simulink model "MPC_AVC_implementation"  (Simulink 7.1)
settings: Solver=ode5  StartTime=0.0  StopTime=Total_t_sim  FixedStep=dt  RelTol=1e-3
PostLoadFcn:
  | , if any(exist('dsrtsu_mdlpostloadfcn', 'file') == [2, 3, 6]), try dsrtsu_mdlpostloadfcn('Execute', bdroot); catch fprintf('Error in PostLoadFcn (dsrtsu_mdlpostloadfcn) for model "%s":\n %s\n', bdroot, lasterr); end, end,
undefined symbols (not defined in the file or in its folder): A, A_cons, Ag, B, Bg, C, coefs, dt, Hg, L_m, Lf, omega, Ps, psi, Rs, Total_t_sim, u_bound
libraries: simulink x3, dsparch4 x1, rti2004lib x1, rtilibm x1
settings Model: Creator=durranbm  LastModifiedBy=oveisahw  BufferReuse=off  DSRTSU_INTERNAL_RTI_VER=330  DSRTSU_INTERNAL_RTI_TYPE=rti1005
settings SolverCC: AlgebraicLoopSolver=LineSearch
settings OptimizationCC: BlockReduction=off  OptimizeBlockIOStorage=off  BufferReuse=off  ExpressionFolding=off  LocalBlockOutputs=off
settings DebuggingCC: AlgebraicLoopMsg=none  ArtificialAlgebraicLoopMsg=none
settings HardwareCC: ProdIntDivRoundTo=Zero  ProdEndianess=BigEndian  ProdHWDeviceType=Specified  TargetIntDivRoundTo=Zero  TargetEndianess=BigEndian
settings RTWCC: SystemTargetFile=rti1005.tlc  MakeCommand=make_rti  TemplateMakefile=rti1005.tmf  Description=dSPACE DS1005 Hardware Platform  ProcessScript=rti1005_make_rtw_hook
settings STFCustomTargetCC: SystemTargetFile=rti1005.tlc
settings GRTTargetCC: CompOptLevelCompliant=off  MatFileLogging=off  ExtModeMexFile=noextcomm
settings CustomProperty: DataType=RTWOptions_EnumType_C__dSPACE_matlab_rti1005_tlc_rti1005_InitialSimState  Value=RUN
settings EnumStrPairs: String=RUN

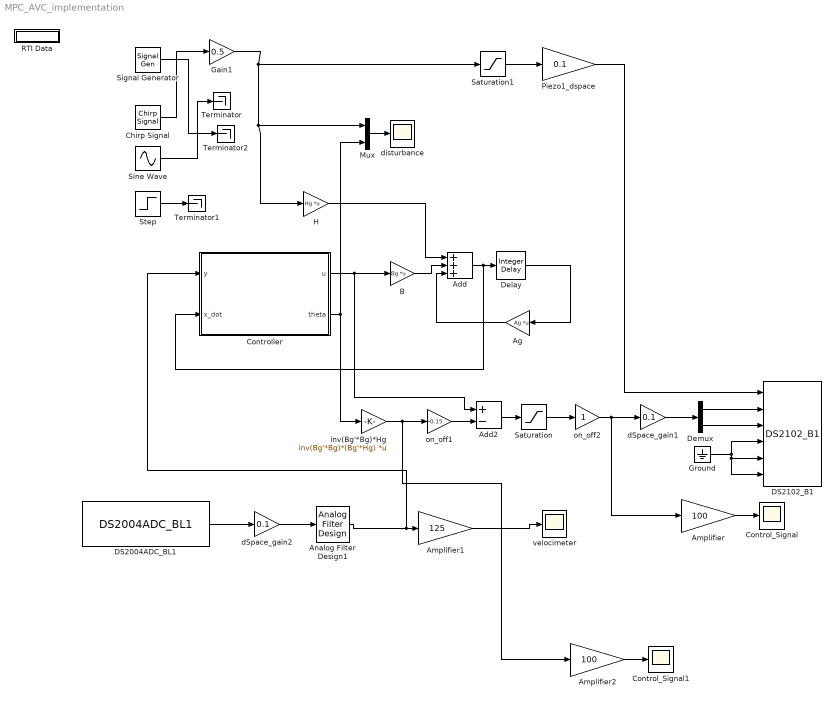
== system MPC_AVC_implementation ==
  Add : Sum  Inputs=+++
  Add2 : Sum  Inputs=+-
  Ag : Gain  Orientation=left  Gain=Ag  Multiplication=Matrix(K*u)
  Amplifier : Gain  Gain=100  ParameterDataType=sfix(16)  ParameterScaling=2^0  OutDataType=sfix(16)  OutScaling=2^0
  Amplifier1 : Gain  Gain=125  ParameterDataType=sfix(16)  ParameterScaling=2^0  OutDataType=sfix(16)  OutScaling=2^0
  Amplifier2 : Gain  Gain=100  ParameterDataType=sfix(16)  ParameterScaling=2^0  OutDataType=sfix(16)  OutScaling=2^0
  Analog Filter Design1 : dsparch4/Analog Filter Design  method=Butterworth  filttype=Lowpass  N=4  Wlo=(2*pi)*400  Whi=80  Rp=2  Rs=40
  B : Gain  Gain=Bg  Multiplication=Matrix(K*u)
  Chirp Signal : simulink/Sources/Chirp Signal  SystemSampleTime=-1  f1=1  T=Total_t_sim  f2=90
  Control_Signal : Scope
      settings: YMin=-1  YMax=1  SaveName=ScopeData2  MaxDataPoints=500000
  Control_Signal1 : Scope
      settings: YMin=-1  YMax=1  SaveName=ScopeData3  MaxDataPoints=500000
  Controller : Subsystem
  DS2004ADC_BL1 : rti2004lib/DS2004ADC_BL1  SystemSampleTime=-1  DSProperties=struct('RTI',struct('Version',uint32(1),'BlockType',struct('isSLSource',uint8(1),'isSLSink',uint8(1),'isHWSource',uint8(0),'isHWSink',uint8(1),'isSetup',uint8(0),'isInline',uint8(1),'isNonInline',uint8(0),'isInterrupt',uint8(0),'isChannelwise',uint8(1)),'IOBoardType','DS2004','UnitType','ADC','Identifier','ADC','DialogType','ML','BlockSet','NONE','SlaveProcessor','NONE'))  RTIBlockInterface=struct('InputPortsActive',0,'InputPortsWidth',int32(1),'InputPortsDataType',{{'SS_BOOLEAN'}},'InputPortsName',{{'Continue'}},'OutputPortsActive',[1 0],'OutputPortsWidth',int32([1 1]),'OutputPortsDataType',{{'SS_DOUBLE','SS_UINT8'}},'OutputPortsName',{{'ADC','Status'}},'DialogFcn','rti2004adcgui','SampleTime',{{-1}},'InitLevel',3,'IconTransparency','on','BlockDisplay',{{['DS2004 ADC\nBoard: 1\nChannel: 1'],'center'}},'BlockName',struct('Token',{{'DS2004ADC_BL1'}}))  RTIBlockParameters=struct('ADCSWStartDisable',{{0,'OFF',[0 1]}},'BoardNo',{{1,'OFF',[1 16]}},'ChannelNo',{{1,'OFF',[1 16]}},'ConversionMode',{{1,'OFF',[1 2]}},'SampleMode',{{1,'OFF',[1 2]}},'TriggerSource',{{1,'OFF',[1 5]}},'EdgePolarity',{{1,'OFF',[1 2]}},'ConversionTriggerSource',{{2,'OFF',[1 6]}},'ConversionEdgePolarity',{{1,'OFF',[1 2]}},'ConversionPeriod',{{'1e-006','OFF',[]}},'ConversionPeriodCheck',{{0,'OFF',[]}},'BurstTriggerSource',{{1,'OFF',[1 6]}},'BurstEdgePolarity',{{1,'OFF',[1 2]}},'BurstSize',{{'10','OFF',[]}},'BurstSizeCheck',{{0,'OFF',[]}},'DataSetOffset',{{'0','OFF',[]}},'DataSetOffsetCheck',{{0,'OFF',[]}},'DataSetLength',{{'1','OFF',[]}},'DataSetLengthCheck',{{0,'OFF',[]}},'ReadMode',{{1,'OFF',[1 2]}},'SampleTime',{{'-1','OFF',[-1 inf]}},'SampleTimeCheck',{{1,'OFF',[]}},'InputVoltageRange',{{2,'OFF',[1 2]}},'StatusPortEnable',{{0,'OFF',[0 1]}},'TLCFileName',{{'rti2004adc','OFF',[]}})  RTISFcnParameters=struct('ADCSWStartDisable','int32','BoardNo','int32','ChannelNo','int32','ConversionMode','int32','SampleMode','int32','TriggerSource','int32','EdgePolarity','int32','ConversionTriggerSource','int32','ConversionEdgePolarity','int32','ConversionPeriod','double','BurstTriggerSource','int32','BurstEdgePolarity','int32','BurstSize','int32','DataSetOffset','int32','DataSetLength','int32','ReadMode','int32','SampleTime','double','InputVoltageRange','int32','StatusPortEnable','int32','TLCFileName','char')  RTIBlockParaDefault=struct('ADCSWStartDisable',0,'BoardNo',1,'ChannelNo',1,'ConversionMode',1,'SampleMode',1,'TriggerSource',1,'EdgePolarity',1,'ConversionTriggerSource',2,'ConversionEdgePolarity',1,'ConversionPeriod',1e-06,'ConversionPeriodCheck',0,'BurstTriggerSource',1,'BurstEdgePolarity',1,'BurstSize',10,'BurstSizeCheck',0,'DataSetOffset',0,'DataSetOffsetCheck',0,'DataSetLength',1,'DataSetLengthCheck',0,'ReadMode',1,'SampleTime',-1,'SampleTimeCheck',1,'InputVoltageRange',2,'StatusPortEnable',0,'TLCFileName','rti2004adc')
  DS2102_B1 : rtilibm/DS2102/DS2102_B1  SystemSampleTime=-1  BoardNo=1  Range=[10 10 10 10 10 10]  IOErrorMode=[1 1 1 1 1 1]  DeglitcherMode=[0 0 0 0 0 0]  InitValue=[0 0 0 0 0 0]  TermMode=[1 1 1 1 1 1]  TermValue=[0 0 0 0 0 0]  DialogFcn=gui2102  UnitName={'DS2102_B'}  UnitValues={ 1 }  DSProperties=struct('RTI',struct('Version',uint32(1),'BlockType',struct('isSLSource',uint8(0),'isSLSink',uint8(1),'isHWSource',uint8(0),'isHWSink',uint8(1),'isSetup',uint8(0),'isInline',uint8(1),'isNonInline',uint8(0),'isInterrupt',uint8(0),'isChannelwise',uint8(0)),'IOBoardType','DS2102','UnitType','DAC','Identifier','DAC','DialogType','ML','BlockSet','NONE','SlaveProcessor','NONE'))
  Delay : simulink/Discrete/Integer Delay  vinit=0  samptime=-1  NumDelays=1
  Demux : Demux  Outputs=2
  Gain1 : Gain  Gain=0.5  ParameterDataType=sfix(16)  ParameterScaling=2^0  OutDataType=sfix(16)  OutScaling=2^0
  Ground : Ground
  H : Gain  Gain=Hg  Multiplication=Matrix(K*u)
  Mux : Mux  Inputs=2
  Piezo1_dspace : Gain  Gain=0.1  ParameterDataType=sfix(16)  ParameterScaling=2^0  OutDataType=sfix(16)  OutScaling=2^0
  RTI Data : Subsystem  Tag=struct('RTIDataServer',struct('RTIDataServerVs','2','RTIModelDescription','struct(''main'',''MPC_AVC_implementation'',''sub'','''',''isMp'',0)'))  LoadFcn="if exist('rtidc'), try,  rtidc('DataHostBlockClbLoad', gcbh); catch, disp(['Warning: ''LoadFcn'' for RTI Data block failed: ' lasterr]); end, end,"
      settings: CopyFcn="if exist('rtidc'), try,  rtidc('DataHostBlockClbCopy', gcbh); catch, disp(['Warning: ''CopyFcn'' for RTI Data block failed: ' lasterr]); end, end,"  DeleteFcn="if exist('rtidc'), try,  rtidc('DataHostBlockClbDelete', gcbh); catch, disp(['Warning: ''DeleteFcn'' for RTI Data block failed: ' lasterr]); end, end,"  ModelCloseFcn="if exist('rtidc'), try,  rtidc('DataHostBlockClbModelClose', gcbh); catch, disp(['Warning: ''ModelCloseFcn'' for RTI Data block failed: ' lasterr]); end, end,"  PreSaveFcn="if exist('rtidc'), try,  rtidc('DataHostBlockClbPreSave', gcbh); catch, disp(['Warning: ''PreSaveFcn'' for RTI Data block failed: ' lasterr]); end, end,"  PostSaveFcn="if exist('rtidc'), try,  rtidc('DataHostBlockClbPostSave', gcbh); catch, disp(['Warning: ''PostSaveFcn'' for RTI Data block failed: ' lasterr]); end, end,"  NameChangeFcn="if exist('rtidc'), try,  rtidc('DataHostBlockClbNameChange', gcbh); catch, disp(['Warning: ''NameChangeFcn'' for RTI Data block failed: ' lasterr]); end, end,"
      mask Type: RTI_DATA_HOST
      mask Description:
      | RTI Data Block.
      | This block is used by RTI to store internal model-dependent data.
      | Please keep this block on the root level of the model. Deleting this block will result in data loss.
      | 
      | NEVER DELETE OR COPY THIS BLOCK!
      mask Help:
      | RTI Data Block.
      | This block is used by RTI to store internal model-dependent data.
      | Please keep this block on the root level of the model. Deleting this block will result in data loss.
      | 
      | NEVER DELETE OR COPY THIS BLOCK!
      mask Display:
      | text(0.5, 0.5, 'RTI Data', 'HorizontalAlignment', 'center');
      | plot([1 0]);
  Saturation : Saturate  UpperLimit=2  LowerLimit=-2  OutDataType=sfix(16)  OutScaling=2^0
  Saturation1 : Saturate  UpperLimit=1  LowerLimit=-1  OutDataType=sfix(16)  OutScaling=2^0
  Signal Generator : SignalGenerator  WaveForm=square  Frequency=1/2.5
  Sine Wave : Sin  Frequency=71*2*pi  SampleTime=dt
  Step : Step  Time=2*dt  SampleTime=0
  Terminator : Terminator
  Terminator1 : Terminator
  Terminator2 : Terminator
  dSpace_gain1 : Gain  Gain=0.1  ParameterDataType=sfix(16)  ParameterScaling=2^0  OutDataType=sfix(16)  OutScaling=2^0
  dSpace_gain2 : Gain  Gain=0.1  ParameterDataType=sfix(16)  ParameterScaling=2^0  OutDataType=sfix(16)  OutScaling=2^0
  disturbance : Scope
      settings: YMin=-0.0007  YMax=0.0007  SaveName=ScopeData5
  inv(Bg'*Bg)*Hg : Gain  Gain=inv(Bg'*Bg)*(Bg'*Hg)  Multiplication=Matrix(K*u)
  on_off1 : Gain  Gain=-0.15
  on_off2 : Gain
  velocimeter : Scope
  wires:
  DS2004ADC_BL1/1 -> dSpace_gain2/1
  dSpace_gain2/1 -> Analog Filter Design1/1
  Amplifier/1 -> Control_Signal/1
  Saturation/1 -> on_off2/1
  on_off2/1 -> Amplifier/1, dSpace_gain1/1
  Step/1 -> Terminator1/1
  dSpace_gain1/1 -> Demux/1
  Demux/1 -> DS2102_B1/2
  Demux/2 -> DS2102_B1/3
  Ground/1 -> DS2102_B1/5, DS2102_B1/6, DS2102_B1/4
  Saturation1/1 -> Piezo1_dspace/1
  Piezo1_dspace/1 -> DS2102_B1/1
  Controller/1(u) -> B/1, Add2/1
  Delay/1 -> Ag/1
  Add/1 -> Controller/2(x_dot), Delay/1
  Ag/1 -> Add/3
  H/1 -> Add/1
  B/1 -> Add/2
  Add2/1 -> Saturation/1
  inv(Bg'*Bg)*Hg/1 -> Amplifier2/1, on_off1/1
  Amplifier1/1 -> velocimeter/1
  Controller/2(theta) -> inv(Bg'*Bg)*Hg/1, Mux/2
  Analog Filter Design1/1 -> Controller/1(y), Amplifier1/1
  Amplifier2/1 -> Control_Signal1/1
  on_off1/1 -> Add2/2
  Sine Wave/1 -> Terminator/1
  Mux/1 -> disturbance/1
  Signal Generator/1 -> Terminator2/1
  Chirp Signal/1 -> Gain1/1
  Gain1/1 -> Saturation1/1, H/1, Mux/1

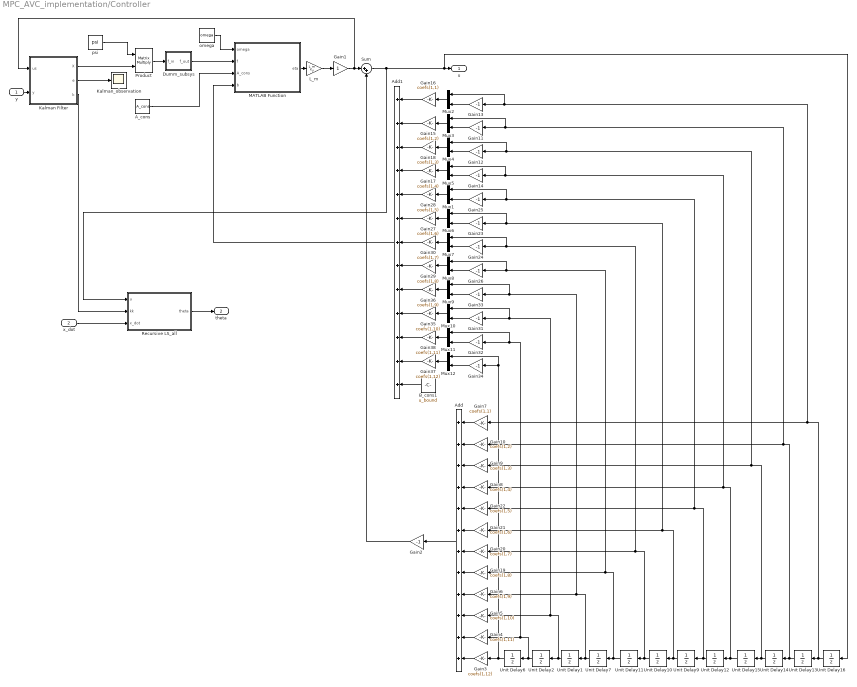
== system MPC_AVC_implementation/Controller ==
  y : Inport
  x_dot : Inport  Port=2
  A_cons : Constant  Value=A_cons  SampleTime=dt
  Add : Sum  Orientation=left  Inputs=++++++++++++
  Add1 : Sum  Orientation=left  Inputs=+++++++++++++
  B_cons1 : Constant  Orientation=left  Value=u_bound
  Dumm_subsys : Subsystem
  Gain1 : Gain
  Gain10 : Gain  Orientation=left  Gain=coefs(1,2)
  Gain{2,11..14,23..26,31..34} (13 alike) : Gain  Orientation=left  Gain=-1
  Gain15 : Gain  Orientation=left  Gain=coefs(1,2)
  Gain16 : Gain  Orientation=left  Gain=coefs(1,1)
  Gain17 : Gain  Orientation=left  Gain=coefs(1,4)
  Gain18 : Gain  Orientation=left  Gain=coefs(1,3)
  Gain19 : Gain  Orientation=left  Gain=coefs(1,8)
  Gain20 : Gain  Orientation=left  Gain=coefs(1,7)
  Gain21 : Gain  Orientation=left  Gain=coefs(1,6)
  Gain22 : Gain  Orientation=left  Gain=coefs(1,5)
  Gain27 : Gain  Orientation=left  Gain=coefs(1,6)
  Gain28 : Gain  Orientation=left  Gain=coefs(1,5)
  Gain29 : Gain  Orientation=left  Gain=coefs(1,8)
  Gain3 : Gain  Orientation=left  Gain=coefs(1,12)
  Gain30 : Gain  Orientation=left  Gain=coefs(1,7)
  Gain35 : Gain  Orientation=left  Gain=coefs(1,10)
  Gain36 : Gain  Orientation=left  Gain=coefs(1,9)
  Gain37 : Gain  Orientation=left  Gain=coefs(1,12)
  Gain38 : Gain  Orientation=left  Gain=coefs(1,11)
  Gain4 : Gain  Orientation=left  Gain=coefs(1,11)
  Gain5 : Gain  Orientation=left  Gain=coefs(1,10)
  Gain6 : Gain  Orientation=left  Gain=coefs(1,9)
  Gain7 : Gain  Orientation=left  Gain=coefs(1,1)
  Gain8 : Gain  Orientation=left  Gain=coefs(1,4)
  Gain9 : Gain  Orientation=left  Gain=coefs(1,3)
  Kalman Filter : Subsystem  TreatAsAtomicUnit=on
      settings: MinAlgLoopOccurrences=on
  Kalman_observation : Scope
      settings: YMin=-0.000155  YMax=-6.5e-05  DataFormat=Array
  L_m : Gain  Gain=L_m  Multiplication=Matrix(K*u)
  MATLAB Function : Stateflow chart  TreatAsAtomicUnit=on
      settings: MinAlgLoopOccurrences=on
  Mux{1..12} (12 alike) : Mux  Orientation=left  Inputs=2
  Product : Product  Multiplication=Matrix(*)  RndMeth=Zero
  Recursive LS_all : Subsystem  TreatAsAtomicUnit=on
      settings: MinAlgLoopOccurrences=on
  Sum : Sum  Inputs=|++
  Unit Delay{1..2,6..7,9..16} (12 alike) : UnitDelay  Orientation=left  SampleTime=dt
  omega : Constant  Value=omega  SampleTime=dt
  psi : Constant  Value=psi  SampleTime=dt
  u : Outport
  theta : Outport  Port=2
  wires:
  MATLAB Function/1(eta) -> L_m/1
  L_m/1 -> Gain1/1
  omega/1 -> MATLAB Function/1(omega)
  A_cons/1 -> MATLAB Function/3(A_cons)
  psi/1 -> Product/1
  y/1 -> Kalman Filter/2(y)
  Gain7/1 -> Add/1
  Gain9/1 -> Add/3
  Gain8/1 -> Add/4
  Gain13/1 -> Mux2/2
  Gain11/1 -> Mux3/2
  Gain12/1 -> Mux4/2
  Gain14/1 -> Mux5/2
  Mux2/1 -> Gain16/1
  Mux3/1 -> Gain15/1
  Mux4/1 -> Gain18/1
  Mux5/1 -> Gain17/1
  Gain16/1 -> Add1/1
  Gain15/1 -> Add1/2
  Gain18/1 -> Add1/3
  Gain17/1 -> Add1/4
  Add/1 -> Gain2/1
  Gain10/1 -> Add/2
  Product/1 -> Dumm_subsys/1(f_in)
  Dumm_subsys/1(f_out) -> MATLAB Function/2(f)
  Kalman Filter/1(X) -> Product/2
  Kalman Filter/2(e) -> Kalman_observation/1
  Gain1/1 -> Sum/1, Kalman Filter/1(us)
  Unit Delay2/1 -> Mux11/1, Gain32/1, Gain4/1, Unit Delay6/1
  Unit Delay1/1 -> Mux10/1, Gain31/1, Gain5/1, Unit Delay2/1
  Unit Delay7/1 -> Gain6/1, Mux9/1, Gain33/1, Unit Delay1/1
  Unit Delay11/1 -> Mux8/1, Gain26/1, Gain19/1, Unit Delay7/1
  Unit Delay10/1 -> Mux7/1, Gain24/1, Gain20/1, Unit Delay11/1
  Unit Delay9/1 -> Mux6/1, Gain23/1, Gain21/1, Unit Delay10/1
  Unit Delay12/1 -> Mux1/1, Gain25/1, Gain22/1, Unit Delay9/1
  Unit Delay15/1 -> Gain14/1, Mux5/1, Gain8/1, Unit Delay12/1
  Unit Delay14/1 -> Mux4/1, Gain12/1, Gain9/1, Unit Delay15/1
  Unit Delay13/1 -> Mux3/1, Gain11/1, Gain10/1, Unit Delay14/1
  Unit Delay16/1 -> Mux2/1, Gain13/1, Gain7/1, Unit Delay13/1
  Gain3/1 -> Add/12
  Unit Delay6/1 -> Gain34/1, Mux12/1, Gain3/1
  Gain4/1 -> Add/11
  Gain5/1 -> Add/10
  Gain6/1 -> Add/9
  Gain19/1 -> Add/8
  Gain20/1 -> Add/7
  Gain21/1 -> Add/6
  Gain22/1 -> Add/5
  B_cons1/1 -> Add1/13
  Gain25/1 -> Mux1/2
  Gain23/1 -> Mux6/2
  Gain24/1 -> Mux7/2
  Gain26/1 -> Mux8/2
  Mux1/1 -> Gain28/1
  Mux6/1 -> Gain27/1
  Mux7/1 -> Gain30/1
  Mux8/1 -> Gain29/1
  Gain33/1 -> Mux9/2
  Gain31/1 -> Mux10/2
  Gain32/1 -> Mux11/2
  Gain34/1 -> Mux12/2
  Mux9/1 -> Gain36/1
  Mux10/1 -> Gain35/1
  Mux11/1 -> Gain38/1
  Mux12/1 -> Gain37/1
  Gain28/1 -> Add1/5
  Gain27/1 -> Add1/6
  Gain30/1 -> Add1/7
  Gain29/1 -> Add1/8
  Gain36/1 -> Add1/9
  Gain35/1 -> Add1/10
  Gain38/1 -> Add1/11
  Gain37/1 -> Add1/12
  Sum/1 -> Recursive LS_all/1(u), Unit Delay16/1, u/1
  Add1/1 -> MATLAB Function/4(b)
  Gain2/1 -> Sum/2
  Recursive LS_all/1(theta) -> theta/1
  x_dot/1 -> Recursive LS_all/3(x_dot)
  Kalman Filter/3(k) -> Recursive LS_all/2(kk)

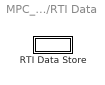
== system MPC_AVC_implementation/RTI Data ==
  RTI Data Store : Subsystem  Tag="struct('private',struct('version',struct('dsVer',uint32(2),'dsVerCreation',uint32(2),'RTI',struct('ver','6.2','type','RTI1005')),'access',struct('type','Model','isPerm',1,'created',['17-Nov-2010 16:10:19'],'modified',['02-Mar-2016 13:36:28'],'location','')),'public',struct('main',struct('data',[]),'sub',struct('name',{{'MPC_AVC_implementation'}},'data',{{struct('TH',struct('thTaskInfo',struct('taskType',{'TIMER','HWINT','TMRINT','SWINT'},'tasksNumOf',{1,0,0,0},'srcIds',{{'TIMERA'},{},{},{}},'entryPoints',{{'rti_TIMERA'},{},{},{}},'taskNames',{{['Timer Task 1']},{},{},{}})),'th_tc',struct('dataType','TASK','taskGroupId','','taskGroupList',{{}},'taskSchedulingPolicy','FCFS','taskType','TIMER','blkh',-1,'srcId','TIMERA','srcSgnName',['Timer A interrupt'],'srcCpuName','','taskName',['Timer Task 1  [0.001] s'],'taskNameDisplayExt','','smplTime',0.001,'smplTimeOffs',0,'hasFixedPriority',0,'priority',1,'hasFixedOvc',0,'ovcType',1,'ovcMax',1),'tc_th',struct('dataType','TASK','taskGroupId','','taskGroupList',{{}},'taskSchedulingPolicy','FCFS','taskType','TIMER','blkh',-1,'srcId','TIMERA','srcSgnName',['Timer A interrupt'],'srcCpuName','','taskName',['Timer Task 1  [0.001] s'],'taskNameDisplayExt','','smplTime',0.001,'smplTimeOffs',0,'hasFixedPriority',0,'priority',1,'hasFixedOvc',0,'ovcType',1,'ovcMax',1))}})))"
      mask Type: RTI_DATA_STORE
      mask Description:
      | RTI Data Store Block. This block is used by RTI to store internal model dependent data. Deleting this block will result in data loss.
      | 
      | NEVER DELETE, COPY, OR MODIFY THIS BLOCK!
      mask Help:
      | RTI Data Store Block. This block is used by RTI to store internal model dependent data. Deleting this block will result in data loss.
      | 
      | NEVER DELETE, COPY, OR MODIFY THIS BLOCK!
      mask Display: text(0.5, 0.5, ' ', 'HorizontalAlignment', 'center');

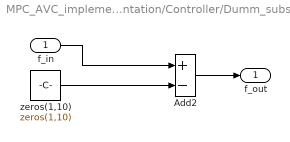
== system MPC_AVC_implementation/Controller/Dumm_subsys ==
  f_in : Inport
  Add2 : Sum  Inputs=+-
  zeros(1,10) : Constant  Value=zeros(1,10)  SampleTime=dt
  f_out : Outport
  wires:
  f_in/1 -> Add2/1
  Add2/1 -> f_out/1
  zeros(1,10)/1 -> Add2/2

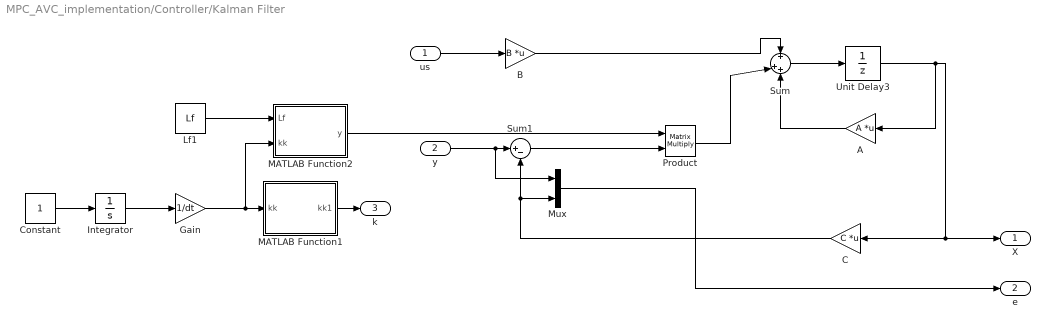
== system MPC_AVC_implementation/Controller/Kalman Filter ==
  us : Inport
  y : Inport  Port=2
  A : Gain  Orientation=left  Gain=A  Multiplication=Matrix(K*u)
  B : Gain  Gain=B  Multiplication=Matrix(K*u)
  C : Gain  Orientation=left  Gain=C  Multiplication=Matrix(K*u)
  Constant : Constant
  Gain : Gain  Gain=1/dt
  Integrator : Integrator
  Lf1 : Constant  Value=Lf
  MATLAB Function1 : Stateflow chart  TreatAsAtomicUnit=on
      settings: MinAlgLoopOccurrences=on
  MATLAB Function2 : Stateflow chart  TreatAsAtomicUnit=on
      settings: MinAlgLoopOccurrences=on
  Mux : Mux  Inputs=2
  Product : Product  Multiplication=Matrix(*)  RndMeth=Zero
  Sum : Sum  Inputs=+|++
  Sum1 : Sum  Inputs=|+-
  Unit Delay3 : UnitDelay  SampleTime=dt
  X : Outport
  e : Outport  Port=2
  k : Outport  Port=3
  wires:
  Unit Delay3/1 -> A/1, X/1, C/1
  A/1 -> Sum/3
  Sum/1 -> Unit Delay3/1
  us/1 -> B/1
  B/1 -> Sum/1
  C/1 -> Mux/2, Sum1/2
  y/1 -> Mux/1, Sum1/1
  Sum1/1 -> Product/2
  Product/1 -> Sum/2
  Lf1/1 -> MATLAB Function2/1(Lf)
  Mux/1 -> e/1
  MATLAB Function2/1(y) -> Product/1
  Constant/1 -> Integrator/1
  Integrator/1 -> Gain/1
  Gain/1 -> MATLAB Function1/1(kk), MATLAB Function2/2(kk)
  MATLAB Function1/1(kk1) -> k/1

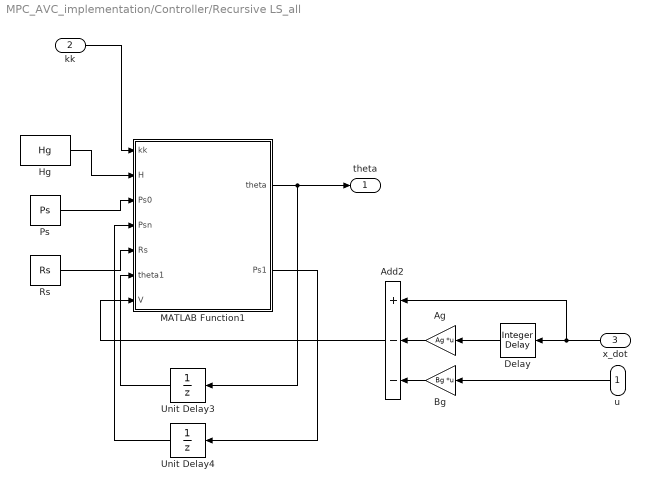
== system MPC_AVC_implementation/Controller/Recursive LS_all ==
  u : Inport  Orientation=left
  kk : Inport  Port=2
  x_dot : Inport  Orientation=left  Port=3
  Add2 : Sum  Orientation=left  Inputs=+--
  Ag : Gain  Orientation=left  Gain=Ag  Multiplication=Matrix(K*u)
  Bg : Gain  Orientation=left  Gain=Bg  Multiplication=Matrix(K*u)
  Delay : simulink/Discrete/Integer Delay  Orientation=left  vinit=0  samptime=-1  NumDelays=1
  Hg : Constant  Value=Hg  SampleTime=dt
  MATLAB Function1 : Stateflow chart  TreatAsAtomicUnit=on
      settings: MinAlgLoopOccurrences=on
  Ps : Constant  Value=Ps  SampleTime=dt
  Rs : Constant  Value=Rs  SampleTime=dt
  Unit Delay3 : UnitDelay  Orientation=left  SampleTime=dt
  Unit Delay4 : UnitDelay  Orientation=left  SampleTime=dt
  theta : Outport
  wires:
  MATLAB Function1/2(Ps1) -> Unit Delay4/1
  MATLAB Function1/1(theta) -> theta/1, Unit Delay3/1
  kk/1 -> MATLAB Function1/1(kk)
  Ps/1 -> MATLAB Function1/3(Ps0)
  Unit Delay3/1 -> MATLAB Function1/6(theta1)
  Hg/1 -> MATLAB Function1/2(H)
  Rs/1 -> MATLAB Function1/5(Rs)
  Unit Delay4/1 -> MATLAB Function1/4(Psn)
  x_dot/1 -> Add2/1, Delay/1
  Delay/1 -> Ag/1
  Ag/1 -> Add2/2
  Bg/1 -> Add2/3
  u/1 -> Bg/1
  Add2/1 -> MATLAB Function1/7(V)

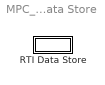
== system MPC_AVC_implementation/RTI Data/RTI Data Store ==
  RTI Data Store : Subsystem
      mask Type: RTI_DATA_STORE
      mask Description:
      | RTI Data Store Block. This block is used by RTI to store internal model dependent data. Deleting this block will result in data loss.
      | 
      | NEVER DELETE, COPY, OR MODIFY THIS BLOCK!
      mask Help:
      | RTI Data Store Block. This block is used by RTI to store internal model dependent data. Deleting this block will result in data loss.
      | 
      | NEVER DELETE, COPY, OR MODIFY THIS BLOCK!
      mask Display: text(0.5, 0.5, ' ', 'HorizontalAlignment', 'center');

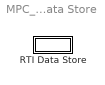
== system MPC_AVC_implementation/RTI Data/RTI Data Store/RTI Data Store ==
  RTI Data Store : Subsystem
      mask Type: RTI_DATA_STORE
      mask Description:
      | RTI Data Store Block. This block is used by RTI to store internal model dependent data. Deleting this block will result in data loss.
      | 
      | NEVER DELETE, COPY, OR MODIFY THIS BLOCK!
      mask Help:
      | RTI Data Store Block. This block is used by RTI to store internal model dependent data. Deleting this block will result in data loss.
      | 
      | NEVER DELETE, COPY, OR MODIFY THIS BLOCK!
      mask Display: text(0.5, 0.5, ' ', 'HorizontalAlignment', 'center');

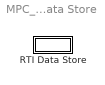
== system MPC_AVC_implementation/RTI Data/RTI Data Store/RTI Data Store/RTI Data Store ==
  RTI Data Store : Subsystem
      mask Type: RTI_DATA_STORE
      mask Description:
      | RTI Data Store Block. This block is used by RTI to store internal model dependent data. Deleting this block will result in data loss.
      | 
      | NEVER DELETE, COPY, OR MODIFY THIS BLOCK!
      mask Help:
      | RTI Data Store Block. This block is used by RTI to store internal model dependent data. Deleting this block will result in data loss.
      | 
      | NEVER DELETE, COPY, OR MODIFY THIS BLOCK!
      mask Display: text(0.5, 0.5, ' ', 'HorizontalAlignment', 'center');

== system MPC_AVC_implementation/RTI Data/RTI Data Store/RTI Data Store/RTI Data Store/RTI Data Store ==

== matlab function Controller/MATLAB Function ==
  data: omega input double; eta output double; f input double; A_cons input double; b input double
function eta=QPomegaild(omega,f,A_cons,b)

[n1,m1]=size(A_cons);
% eta=-omega\f;
eta=-inv(omega)*f;
kk=0;
for i=1:n1
    if (A_cons(i,:)*eta>b(i)) 
        kk=kk+1;
    else
        kk=kk+0;
    end
end
if (kk==0)
    return
end
P=A_cons*(omega\A_cons');
d=(A_cons*(omega\f)+b);
[n,m]=size(d);
x_ini=zeros(n,m);
lambda=x_ini;
% al=10;
for km=1:38

%find tomegae elements in tomegae solution vector one by one
% km could be larger if tomegae Lagranger multiplier omegaas a slow
% convergence rate.
    lambda_p=lambda;
    for i=1:n
        w= P(i,:)*lambda-P(i,i)*lambda(i,1);
        w=w+d(i,1);
        la=-w/P(i,i);
        lambda(i,1)=max(0,la);
    end
    
    al=(lambda-lambda_p)'*(lambda-lambda_p);
    if (al<10e-8)
        break;
    end
 end
eta=-omega\f -omega\A_cons'*lambda;

== matlab function Controller/Kalman Filter/MATLAB Function2 ==
  data: y output double; Lf input double; kk input double
function y = fcn(Lf,kk)
%#eml

kk1 = floor(kk)+1;

y = Lf(:,kk1);

== matlab function Controller/Kalman Filter/MATLAB Function1 ==
  data: kk1 output double; kk input double
function kk1 = fcn(kk)
%#eml

kk1 = floor(kk)+1;

== matlab function Controller/Recursive LS_all/MATLAB Function1 ==
  data: kk input double; H input double; Ps0 input double; Psn input double; Rs input double; theta1 input double; theta output double; Ps1 output double; V input double
function [theta,Ps1] = fcn(kk,H,Ps0,Psn,Rs,theta1,V)
%#eml
if (kk==1)
    Ps = Ps0;
    Ks=(Ps*H')/(H*Ps*H'+Rs);
    theta=theta1+Ks*(V-H*theta1);
    Ps1=(eye(1)-Ks*H)*Ps*(eye(1)-Ks*H)'+Ks*Rs*Ks';
else
    Ps = Psn;
    Ks=(Ps*H')/(H*Ps*H'+Rs);
    theta=theta1+Ks*(V-H*theta1);
    Ps1=(eye(1)-Ks*H)*Ps*(eye(1)-Ks*H)'+Ks*Rs*Ks';
end
